simulink model "CSI_0313_4DC"  (R2018a)
settings: Solver=FixedStepDiscrete  StartTime=0.0  StopTime=Tstop  FixedStep=Tdelt  MaxStep=1e-4  RelTol=1e-3
values from neighbouring files (symbols this model uses):
  C = 12e-6    (= 1.2e-05)    [Inputparameter.m]
  Cdc = 4.76*10^-3    (= 0.00476)    [Inputparameter.m]
  Cemc = 1.5e-6    (= 1.5e-06)    [Inputparameter.m]
  fanalog = 7000    [Run.m]
  fKIUdc = 6    [Run.m]
  fKPUdc = 0.4    [Run.m]
  fTs = Update/18000    (= 0.000111111111111)    [Run.m]
  K120 = 0.0    (= 0)    [Run.m]
  K21 = 0.0    (= 0)    [Run.m]
  K5 = 0.0    (= 0)    [Run.m]
  K7 = 0.0    (= 0)    [Run.m]
  Kipll = 1.0    (= 1)    [Run.m]
  klmt = 0.3    [Run.m]
  Kpll = 20.0    (= 20)    [Run.m]
  Lgrid = 7.717e-4*10    (= 0.007717)    [Run.m]
  Lline = 60e-6    (= 6e-05)    [Inputparameter.m]
  Lpwm = 184.8e-6    (= 0.0001848)    [Inputparameter.m]
  mode = 1    [Run.m]
  Nsw = 18000/fbase    [Run.m]
  Qbpf = 1.0    (= 1)    [Run.m]
  Rc = 10e-3    (= 0.01)    [Inputparameter.m]
  Remc = 1e-3    (= 0.001)    [Inputparameter.m]
  Rgrid = 2*pi*fbase*Lgrid/XR    [Run.m]
  Rline = 4.95e-3    (= 0.00495)    [Inputparameter.m]
  Rpre = 2.2    [Inputparameter.m]
  Rpwm = 6.2e-3    (= 0.0062)    [Inputparameter.m]
  Tdelt = (fTs)/(200*Update)    (= 2.77777777778e-07)    [Run.m]
  Tdt = 1.27e-6    (= 1.27e-06)    [Run.m]
  tstart = 0.2    [Run.m]
  Tvstep = 1.5    [Run.m]
  Update = 2    [Run.m]
  Vbase = 400*sqrt(2/3)    [Inputparameter.m]
undefined symbols (not defined in the file or in its folder): sigbuilder_block
libraries: powerlib x412
(part 4 of 13)

== system CSI_0313_4DC/AIP2/Subsystem5 ==
  Vabc : Inport
  Trigger : TriggerPort  TriggerType=falling  VariantControl=Variant  PortDimensions=1
  Gain6 : Gain  Gain=1/Vbase
  PLL : Subsystem  mask{fKPPLL=Kpll, fKIPLL=Kipll, fDltMin=-19, fDltMax=19, fFqBase=50, fTs=fTs}
      mask prompts: fKPPLL "PLL Proportional Gain"; fKIPLL "PLL Integral Coefficient"; fDltMin "fDelta Minimum Limitation [rad/s]"; fDltMax "fDelta Maximum Limitation [rad/s]"; fFqBase "Base Frequency [Hz]"; fTs "Sample Time [s]"
  Freq : Outport
  wt : Outport  Port=2
  VdPosPU : Outport  Port=3
  wires:
  Gain6/1 -> [VabcPU]
  PLL/2(wt) -> wt/1
  Vabc/1 -> Gain6/1
  [VabcPU] -> PLL/1(Vabc)
  PLL/3(VdPos) -> VdPosPU/1
  PLL/1(f) -> Freq/1

== system CSI_0313_4DC/AIP2/Subsystem7 ==
  Vpcc : Inport
  Vdcs : Inport  Port=2
  VdcsLP : Inport  Port=3
  "Freq " : Inport  Port=4
  wt : Inport  Port=5
  Enable : EnablePort
  Trigger : TriggerPort  TriggerType=falling  VariantControl=Variant  PortDimensions=1
  ABC_To_RIZ1 : MATLAB Function  TreatAsAtomicUnit=on
  "BPF " : Subsystem
  Gain1 : Gain  Gain=Vbase
  Gain5 : Gain  Gain=1/Vbase
  Pos Compensation1 : Subsystem
  RIZ_To_ABC1 : MATLAB Function  TreatAsAtomicUnit=on
  Scope2 : Scope  NumInputPorts=3
  Scope4 : Scope  NumInputPorts=2
  Subsystem5 : Subsystem
  Sum : Sum
  Vmod : Outport  VectorParamsAs1DForOutWhenUnconnected=on
  wires:
  [VabcBPFPU] -> Sum/2
  Pos Compensation1/1(VabcFBPU) -> [VabcFBPU]
  [wt] -> Pos Compensation1/2(wt)
  [Vdc] -> Pos Compensation1/1(Vdc)
  wt/1 -> [wt], Scope4/2
  "Freq "/1 -> [freq], Scope4/1
  VdcsLP/1 -> [VdcLP]
  Gain5/1 -> [VrizPU]
  [Vriz] -> Gain5/1
  [Vdc] -> Scope2/3
  [VdcLP] -> Subsystem5/2(Vdc)
  Vdcs/1 -> [Vdc]
  [VabcBPFPU] -> Scope2/2
  [VabcFBPU] -> Scope2/1
  Vpcc/1 -> [Vabc]
  [VrizBPFPU] -> RIZ_To_ABC1/1(RIZ)
  ABC_To_RIZ1/1(RIZ) -> [Vriz]
  [Vabc] -> ABC_To_RIZ1/1(ABC)
  [freq] -> "BPF "/2(Freq)
  RIZ_To_ABC1/1(ABC) -> [VabcBPFPU]
  [VrizPU] -> "BPF "/1(Vriz)
  "BPF "/1(VpccBPF) -> [VrizBPFPU]
  [VMod_3rd] -> Vmod/1
  [VabcMod] -> Subsystem5/1(Vabc)
  Gain1/1 -> [VabcMod]
  Sum/1 -> Gain1/1
  Subsystem5/1(Vmod) -> [VMod_3rd]
  [VabcFBPU] -> Sum/1

== system CSI_0313_4DC/AIP3/Cemc ==
  RLemc1 : powerlib/Elements/Series RLC Branch  LConnTagsString=__new0  RConnTagsString=__new0  BranchType=RC  Resistance=Remc  Inductance=Lpwm  SetiL0=off  InitialCurrent=0  Capacitance=Cemc  Setx0=off  InitialVoltage=326.6  Measurements=None
      settings: SourceProductName=Simscape Electrical
  RLemc2 : powerlib/Elements/Series RLC Branch  LConnTagsString=__new0  RConnTagsString=__new0  BranchType=RC  Resistance=Remc  Inductance=Lpwm  SetiL0=off  InitialCurrent=0  Capacitance=Cemc  Setx0=off  InitialVoltage=326.6  Measurements=None
      settings: SourceProductName=Simscape Electrical
  RLemc3 : powerlib/Elements/Series RLC Branch  LConnTagsString=__new0  RConnTagsString=__new0  BranchType=RC  Resistance=Remc  Inductance=Lpwm  SetiL0=off  InitialCurrent=0  Capacitance=Cemc  Setx0=off  InitialVoltage=326.6  Measurements=None
      settings: SourceProductName=Simscape Electrical
  ConnA : PMIOPort  Side=Left
  ConnB : PMIOPort  Port=2  Side=Left
  ConnC : PMIOPort  Port=3  Side=Left
  Gnd : PMIOPort  Port=4  Side=Right
  connections:
  RLemc1/LConn1 -- ConnA/RConn1
  RLemc3/RConn1 -- Gnd/RConn1 -- RLemc1/RConn1 -- RLemc2/RConn1
  RLemc2/LConn1 -- ConnB/RConn1
  RLemc3/LConn1 -- ConnC/RConn1

== system CSI_0313_4DC/AIP3/LCL Output Filter ==
  RL : powerlib/Elements/Series RLC Branch  LConnTagsString=__new0  RConnTagsString=__new0  BranchType=RL  Resistance=Rpwm  Inductance=Lpwm  SetiL0=off  InitialCurrent=0  Capacitance=1e-6  Setx0=off  InitialVoltage=0  Measurements=None
      settings: SourceProductName=Simscape Electrical
  RL1 : powerlib/Elements/Series RLC Branch  LConnTagsString=__new0  RConnTagsString=__new0  BranchType=RL  Resistance=Rpwm  Inductance=Lpwm  SetiL0=off  InitialCurrent=0  Capacitance=1e-6  Setx0=off  InitialVoltage=0  Measurements=None
      settings: SourceProductName=Simscape Electrical
  RL2 : powerlib/Elements/Series RLC Branch  LConnTagsString=__new0  RConnTagsString=__new0  BranchType=RL  Resistance=Rpwm  Inductance=Lpwm  SetiL0=off  InitialCurrent=0  Capacitance=1e-6  Setx0=off  InitialVoltage=0  Measurements=None
      settings: SourceProductName=Simscape Electrical
  RL3 : powerlib/Elements/Series RLC Branch  LConnTagsString=__new0  RConnTagsString=__new0  BranchType=RL  Resistance=Rline  Inductance=Lline  SetiL0=off  InitialCurrent=0  Capacitance=1e-6  Setx0=off  InitialVoltage=0  Measurements=None
      settings: SourceProductName=Simscape Electrical
  RL4 : powerlib/Elements/Series RLC Branch  LConnTagsString=__new0  RConnTagsString=__new0  BranchType=RL  Resistance=Rline  Inductance=Lline  SetiL0=off  InitialCurrent=0  Capacitance=1e-6  Setx0=off  InitialVoltage=0  Measurements=None
      settings: SourceProductName=Simscape Electrical
  RL5 : powerlib/Elements/Series RLC Branch  LConnTagsString=__new0  RConnTagsString=__new0  BranchType=RL  Resistance=Rline  Inductance=Lline  SetiL0=off  InitialCurrent=0  Capacitance=1e-6  Setx0=off  InitialVoltage=0  Measurements=None
      settings: SourceProductName=Simscape Electrical
  RL6 : powerlib/Elements/Series RLC Branch  LConnTagsString=__new0  RConnTagsString=__new0  BranchType=RC  Resistance=Rc  Inductance=Lpwm  SetiL0=off  InitialCurrent=0  Capacitance=C  Setx0=off  InitialVoltage=326.6  Measurements=None
      settings: SourceProductName=Simscape Electrical
  RL7 : powerlib/Elements/Series RLC Branch  LConnTagsString=__new0  RConnTagsString=__new0  BranchType=RC  Resistance=Rc  Inductance=Lpwm  SetiL0=off  InitialCurrent=0  Capacitance=C  Setx0=off  InitialVoltage=326.6  Measurements=None
      settings: SourceProductName=Simscape Electrical
  RL8 : powerlib/Elements/Series RLC Branch  LConnTagsString=__new0  RConnTagsString=__new0  BranchType=RC  Resistance=Rc  Inductance=Lpwm  SetiL0=off  InitialCurrent=0  Capacitance=C  Setx0=off  InitialVoltage=326.6  Measurements=None
      settings: SourceProductName=Simscape Electrical
  ConnA : PMIOPort  Side=Left
  Conna : PMIOPort  Port=2  Side=Right
  ConnB : PMIOPort  Port=3  Side=Left
  Connb : PMIOPort  Port=4  Side=Right
  ConnC : PMIOPort  Port=5  Side=Left
  Connc : PMIOPort  Port=6  Side=Right
  "Neutral " : PMIOPort  Port=7  Side=Right
  connections:
  RL4/LConn1 -- RL7/LConn1 -- RL1/RConn1
  RL/LConn1 -- ConnA/RConn1
  RL3/LConn1 -- RL6/LConn1 -- RL/RConn1
  RL5/LConn1 -- RL8/LConn1 -- RL2/RConn1
  RL4/RConn1 -- Connb/RConn1
  RL6/RConn1 -- RL7/RConn1 -- "Neutral "/RConn1 -- RL8/RConn1
  RL1/LConn1 -- ConnB/RConn1
  RL3/RConn1 -- Conna/RConn1
  RL2/LConn1 -- ConnC/RConn1
  RL5/RConn1 -- Connc/RConn1

== system CSI_0313_4DC/AIP3/RB-IGBT Bridge1 ==
  Gate : Inport
  Demux : Demux
  Demux1 : Demux
  Demux2 : Demux
  Demux3 : Demux  Outputs=3
  IGBT/Diode{1..5,12} (6 alike) : powerlib/Power Electronics/IGBT//Diode  Ron=Ron1  Rs=1e6  Cs=Cout  Measurements=off
      settings: SourceProductName=Simscape Electrical
  IGBT/Diode{6..11} (6 alike) : powerlib/Power Electronics/IGBT//Diode  Ron=Ron2  Rs=1e6  Cs=Cout  Measurements=off
      settings: SourceProductName=Simscape Electrical
  positive : PMIOPort  Tag=PMCPort  Side=Right
  netural : PMIOPort  Tag=PMCPort  Port=2  Side=Right
  negative : PMIOPort  Tag=PMCPort  Port=3  Side=Right
  A : PMIOPort  Tag=PMCPort  Port=4  Side=Left
  B : PMIOPort  Tag=PMCPort  Port=5  Side=Left
  C : PMIOPort  Tag=PMCPort  Port=6  Side=Left
  wires:
  Demux3/3 -> Demux2/1  "PulseC"
  Demux3/2 -> Demux1/1  "PulseB"
  Demux3/1 -> Demux/1  "PulseA"
  [PulseC_2n] -> IGBT/Diode4/1
  Demux2/4 -> [PulseC_2n]
  Demux2/3 -> [PulseC_1n]
  Demux2/2 -> [PulseC_2p]
  Demux2/1 -> [PulseC_1p]
  [PulseB_2n] -> IGBT/Diode3/1
  Demux1/4 -> [PulseB_2n]
  Demux1/3 -> [PulseB_1n]
  [PulseB_2p] -> IGBT/Diode8/1
  Demux1/2 -> [PulseB_2p]
  [PulseB_1p] -> IGBT/Diode1/1
  Demux1/1 -> [PulseB_1p]
  [PulseA_2n] -> IGBT/Diode12/1
  Demux/4 -> [PulseA_2n]
  Demux/3 -> [PulseA_1n]
  [PulseA_2p] -> IGBT/Diode6/1
  Demux/2 -> [PulseA_2p]
  [PulseA_1p] -> IGBT/Diode5/1
  Demux/1 -> [PulseA_1p]
  Gate/1 -> Demux3/1
  [PulseA_1n] -> IGBT/Diode7/1
  [PulseB_1n] -> IGBT/Diode9/1
  [PulseC_2p] -> IGBT/Diode10/1
  [PulseC_1n] -> IGBT/Diode11/1
  [PulseC_1p] -> IGBT/Diode2/1
  connections:
  C/RConn1 -- IGBT/Diode4/LConn1 -- IGBT/Diode2/RConn1 -- IGBT/Diode11/LConn1
  netural/RConn1 -- IGBT/Diode10/LConn1 -- IGBT/Diode8/LConn1 -- IGBT/Diode6/LConn1
  A/RConn1 -- IGBT/Diode12/LConn1 -- IGBT/Diode5/RConn1 -- IGBT/Diode7/LConn1
  B/RConn1 -- IGBT/Diode3/LConn1 -- IGBT/Diode1/RConn1 -- IGBT/Diode9/LConn1
  IGBT/Diode2/LConn1 -- positive/RConn1 -- IGBT/Diode1/LConn1 -- IGBT/Diode5/LConn1
  IGBT/Diode4/RConn1 -- negative/RConn1 -- IGBT/Diode12/RConn1 -- IGBT/Diode3/RConn1
  IGBT/Diode7/RConn1 -- IGBT/Diode6/RConn1
  IGBT/Diode9/RConn1 -- IGBT/Diode8/RConn1
  IGBT/Diode11/RConn1 -- IGBT/Diode10/RConn1

== system CSI_0313_4DC/AIP3/SPWM_Three Level ==
  VMod_3rd : Inport
  Freq : Inport  Port=2
  Tstart : Inport  Port=3
  Carrier Gen : MATLAB Function  TreatAsAtomicUnit=on  mask{fdelt=Tdelt}
      mask prompts: fdelt "Simulation Step [s]"
  Constant1 : Constant  Value=Nsw
  Constant2 : Constant  Value=18000
  Constant3 : Constant  Value=55e-6
  Constant4 : Constant  Value=Update
  Constant6 : Constant  Value=Update
  Delay1 : Delay  DelayLength=1  SampleTime=fTs
  Demux1 : Demux  Outputs=3
  Mux : Mux
  Product1 : Product
  Product2 : Product
  Pulse Modulation : MATLAB Function  TreatAsAtomicUnit=on
  Scope1 : Scope
  Scope2 : Scope  NumInputPorts=5
  Step : Step  Time=tstart  Before=-1  SampleTime=0
  Switch : Switch  Criteria=u2 > Threshold
  Tdt Insert : MATLAB Function  TreatAsAtomicUnit=on  mask{tdt=Tdt, fdelt=Tdelt}
      mask prompts: tdt "Dead Time [s]"; fdelt "Simulation step [s]"
  Voltage update timing generator : MATLAB Function  TreatAsAtomicUnit=on
  Voltage update timing generator1 : MATLAB Function  TreatAsAtomicUnit=on
  Gate : Outport  VectorParamsAs1DForOutWhenUnconnected=on
  Ttrigger : Outport  Port=2  VectorParamsAs1DForOutWhenUnconnected=on
  Ttrigger1 : Outport  Port=3  VectorParamsAs1DForOutWhenUnconnected=on
  chk : Outport  Port=4  VectorParamsAs1DForOutWhenUnconnected=on
  wires:
  Mux/1 -> chk/1
  [chk] -> Mux/4
  [Tupdate] -> Mux/3
  [carrier] -> Mux/1
  Voltage update timing generator/1(Tupdate) -> [Tupdate]
  [Ttrigger] -> Voltage update timing generator/1(Trigger)
  [carrier] -> Pulse Modulation/1(carrier)
  Carrier Gen/1(carrier) -> [carrier]
  Carrier Gen/2(sgn) -> [Ttrigger]
  [Freq] -> Carrier Gen/1(fsw)
  Product2/1 -> Switch/1
  Delay1/1 -> Product2/1
  Constant2/1 -> [Freq], Switch/3
  Constant1/1 -> Product2/2
  Step/1 -> Switch/2
  Freq/1 -> Delay1/1
  [Freq] -> Product1/1
  Product1/1 -> Mux/2
  Constant3/1 -> Product1/2
  Switch/1 -> Scope1/1
  Tstart/1 -> Tdt Insert/2(st)
  [Tupdatex] -> Pulse Modulation/3(update)
  Pulse Modulation/1(Pulse) -> Tdt Insert/1(pulse)
  Constant4/1 -> Voltage update timing generator/2(Update)
  Tdt Insert/1(Gate) -> Gate/1
  Constant6/1 -> Voltage update timing generator1/2(Update)
  [Ttrigger] -> Voltage update timing generator1/1(Trigger)
  [Tupdate] -> Ttrigger1/1
  [Ttrigger] -> Ttrigger/1
  Pulse Modulation/2(chk) -> [chk]
  Voltage update timing generator1/1(Tupdate) -> [Tupdatex]
  [Ttrigger] -> Pulse Modulation/2(sgn)
  VMod_3rd/1 -> [VMod_3rd]
  [VMod_3rd] -> Pulse Modulation/4(mod)
  Pulse Modulation/3(chk1) -> [chk1]
  [Tupdatex] -> Scope2/1
  [Ttrigger] -> Scope2/2
  [VMod_3rd] -> Demux1/1
  Demux1/1 -> Scope2/5
  [chk1] -> Scope2/4
  [Tupdate] -> Scope2/3

== system CSI_0313_4DC/AIP3/Subsystem ==
  In1 : Inport
  Demux2 : Demux  Outputs=3
  IIR_1st1 : MATLAB Function  TreatAsAtomicUnit=on  mask{fc=fanalog, fTs=Tdelt}
      mask prompts: fc "Cut-off frequency [Hz]"; fTs "Sample time [s]"
      mask help: 1st-order Low Pass Filter
  IIR_1st2 : MATLAB Function  TreatAsAtomicUnit=on  mask{fc=fanalog, fTs=Tdelt}
      mask prompts: fc "Cut-off frequency [Hz]"; fTs "Sample time [s]"
      mask help: 1st-order Low Pass Filter
  IIR_1st3 : MATLAB Function  TreatAsAtomicUnit=on  mask{fc=fanalog, fTs=Tdelt}
      mask prompts: fc "Cut-off frequency [Hz]"; fTs "Sample time [s]"
      mask help: 1st-order Low Pass Filter
  Mux1 : Mux  Inputs=3
  Out1 : Outport  VectorParamsAs1DForOutWhenUnconnected=on
  wires:
  IIR_1st2/1(y) -> Mux1/2
  In1/1 -> Demux2/1
  Demux2/1 -> IIR_1st1/1(u)
  Demux2/3 -> IIR_1st3/1(u)
  Demux2/2 -> IIR_1st2/1(u)
  IIR_1st3/1(y) -> Mux1/3
  Mux1/1 -> Out1/1
  IIR_1st1/1(y) -> Mux1/1

== system CSI_0313_4DC/AIP3/Subsystem3 ==
  In1 : Inport
  Trigger : TriggerPort  VariantControl=Variant  PortDimensions=1
  IIR_1st1 : MATLAB Function  TreatAsAtomicUnit=on  mask{fc=10, fTs=fTs}
      mask prompts: fc "Cut-off frequency [Hz]"; fTs "Sample time [s]"
      mask help: 1st-order Low Pass Filter
  Out1 : Outport  VectorParamsAs1DForOutWhenUnconnected=on
  wires:
  IIR_1st1/1(y) -> Out1/1
  In1/1 -> IIR_1st1/1(u)

== system CSI_0313_4DC/AIP3/Subsystem5 ==
  Vabc : Inport
  Trigger : TriggerPort  TriggerType=falling  VariantControl=Variant  PortDimensions=1
  Gain6 : Gain  Gain=1/Vbase
  PLL : Subsystem  mask{fKPPLL=Kpll, fKIPLL=Kipll, fDltMin=-19, fDltMax=19, fFqBase=50, fTs=fTs}
      mask prompts: fKPPLL "PLL Proportional Gain"; fKIPLL "PLL Integral Coefficient"; fDltMin "fDelta Minimum Limitation [rad/s]"; fDltMax "fDelta Maximum Limitation [rad/s]"; fFqBase "Base Frequency [Hz]"; fTs "Sample Time [s]"
  Freq : Outport
  wt : Outport  Port=2
  VdPosPU : Outport  Port=3
  wires:
  PLL/1(f) -> Freq/1
  PLL/3(VdPos) -> VdPosPU/1
  [VabcPU] -> PLL/1(Vabc)
  Vabc/1 -> Gain6/1
  PLL/2(wt) -> wt/1
  Gain6/1 -> [VabcPU]

== system CSI_0313_4DC/AIP3/Subsystem7 ==
  Vpcc : Inport
  Vdcs : Inport  Port=2
  VdcsLP : Inport  Port=3
  "Freq " : Inport  Port=4
  wt : Inport  Port=5
  Enable : EnablePort
  Trigger : TriggerPort  TriggerType=falling  VariantControl=Variant  PortDimensions=1
  ABC_To_RIZ1 : MATLAB Function  TreatAsAtomicUnit=on
  "BPF " : Subsystem
  Gain1 : Gain  Gain=Vbase
  Gain5 : Gain  Gain=1/Vbase
  Pos Compensation1 : Subsystem
  RIZ_To_ABC1 : MATLAB Function  TreatAsAtomicUnit=on
  Scope2 : Scope  NumInputPorts=3
  Scope4 : Scope  NumInputPorts=2
  Subsystem5 : Subsystem
  Sum : Sum
  Vmod : Outport  VectorParamsAs1DForOutWhenUnconnected=on
  wires:
  [VabcFBPU] -> Sum/1
  Subsystem5/1(Vmod) -> [VMod_3rd]
  Sum/1 -> Gain1/1
  Gain1/1 -> [VabcMod]
  [VabcMod] -> Subsystem5/1(Vabc)
  [VMod_3rd] -> Vmod/1
  "BPF "/1(VpccBPF) -> [VrizBPFPU]
  [VrizPU] -> "BPF "/1(Vriz)
  RIZ_To_ABC1/1(ABC) -> [VabcBPFPU]
  [freq] -> "BPF "/2(Freq)
  [Vabc] -> ABC_To_RIZ1/1(ABC)
  ABC_To_RIZ1/1(RIZ) -> [Vriz]
  [VrizBPFPU] -> RIZ_To_ABC1/1(RIZ)
  Vpcc/1 -> [Vabc]
  [VabcFBPU] -> Scope2/1
  [VabcBPFPU] -> Scope2/2
  Vdcs/1 -> [Vdc]
  [VdcLP] -> Subsystem5/2(Vdc)
  [Vdc] -> Scope2/3
  [Vriz] -> Gain5/1
  Gain5/1 -> [VrizPU]
  VdcsLP/1 -> [VdcLP]
  "Freq "/1 -> Scope4/1, [freq]
  wt/1 -> Scope4/2, [wt]
  [Vdc] -> Pos Compensation1/1(Vdc)
  [wt] -> Pos Compensation1/2(wt)
  Pos Compensation1/1(VabcFBPU) -> [VabcFBPU]
  [VabcBPFPU] -> Sum/2

== system CSI_0313_4DC/AIP4/Cemc ==
  RLemc1 : powerlib/Elements/Series RLC Branch  LConnTagsString=__new0  RConnTagsString=__new0  BranchType=RC  Resistance=Remc  Inductance=Lpwm  SetiL0=off  InitialCurrent=0  Capacitance=Cemc  Setx0=off  InitialVoltage=326.6  Measurements=None
      settings: SourceProductName=Simscape Electrical
  RLemc2 : powerlib/Elements/Series RLC Branch  LConnTagsString=__new0  RConnTagsString=__new0  BranchType=RC  Resistance=Remc  Inductance=Lpwm  SetiL0=off  InitialCurrent=0  Capacitance=Cemc  Setx0=off  InitialVoltage=326.6  Measurements=None
      settings: SourceProductName=Simscape Electrical
  RLemc3 : powerlib/Elements/Series RLC Branch  LConnTagsString=__new0  RConnTagsString=__new0  BranchType=RC  Resistance=Remc  Inductance=Lpwm  SetiL0=off  InitialCurrent=0  Capacitance=Cemc  Setx0=off  InitialVoltage=326.6  Measurements=None
      settings: SourceProductName=Simscape Electrical
  ConnA : PMIOPort  Side=Left
  ConnB : PMIOPort  Port=2  Side=Left
  ConnC : PMIOPort  Port=3  Side=Left
  Gnd : PMIOPort  Port=4  Side=Right
  connections:
  RLemc3/LConn1 -- ConnC/RConn1
  RLemc2/LConn1 -- ConnB/RConn1
  RLemc2/RConn1 -- RLemc1/RConn1 -- Gnd/RConn1 -- RLemc3/RConn1
  RLemc1/LConn1 -- ConnA/RConn1

== system CSI_0313_4DC/AIP4/LCL Output Filter ==
  RL : powerlib/Elements/Series RLC Branch  LConnTagsString=__new0  RConnTagsString=__new0  BranchType=RL  Resistance=Rpwm  Inductance=Lpwm  SetiL0=off  InitialCurrent=0  Capacitance=1e-6  Setx0=off  InitialVoltage=0  Measurements=None
      settings: SourceProductName=Simscape Electrical
  RL1 : powerlib/Elements/Series RLC Branch  LConnTagsString=__new0  RConnTagsString=__new0  BranchType=RL  Resistance=Rpwm  Inductance=Lpwm  SetiL0=off  InitialCurrent=0  Capacitance=1e-6  Setx0=off  InitialVoltage=0  Measurements=None
      settings: SourceProductName=Simscape Electrical
  RL2 : powerlib/Elements/Series RLC Branch  LConnTagsString=__new0  RConnTagsString=__new0  BranchType=RL  Resistance=Rpwm  Inductance=Lpwm  SetiL0=off  InitialCurrent=0  Capacitance=1e-6  Setx0=off  InitialVoltage=0  Measurements=None
      settings: SourceProductName=Simscape Electrical
  RL3 : powerlib/Elements/Series RLC Branch  LConnTagsString=__new0  RConnTagsString=__new0  BranchType=RL  Resistance=Rline  Inductance=Lline  SetiL0=off  InitialCurrent=0  Capacitance=1e-6  Setx0=off  InitialVoltage=0  Measurements=None
      settings: SourceProductName=Simscape Electrical
  RL4 : powerlib/Elements/Series RLC Branch  LConnTagsString=__new0  RConnTagsString=__new0  BranchType=RL  Resistance=Rline  Inductance=Lline  SetiL0=off  InitialCurrent=0  Capacitance=1e-6  Setx0=off  InitialVoltage=0  Measurements=None
      settings: SourceProductName=Simscape Electrical
  RL5 : powerlib/Elements/Series RLC Branch  LConnTagsString=__new0  RConnTagsString=__new0  BranchType=RL  Resistance=Rline  Inductance=Lline  SetiL0=off  InitialCurrent=0  Capacitance=1e-6  Setx0=off  InitialVoltage=0  Measurements=None
      settings: SourceProductName=Simscape Electrical
  RL6 : powerlib/Elements/Series RLC Branch  LConnTagsString=__new0  RConnTagsString=__new0  BranchType=RC  Resistance=Rc  Inductance=Lpwm  SetiL0=off  InitialCurrent=0  Capacitance=C  Setx0=off  InitialVoltage=326.6  Measurements=None
      settings: SourceProductName=Simscape Electrical
  RL7 : powerlib/Elements/Series RLC Branch  LConnTagsString=__new0  RConnTagsString=__new0  BranchType=RC  Resistance=Rc  Inductance=Lpwm  SetiL0=off  InitialCurrent=0  Capacitance=C  Setx0=off  InitialVoltage=326.6  Measurements=None
      settings: SourceProductName=Simscape Electrical
  RL8 : powerlib/Elements/Series RLC Branch  LConnTagsString=__new0  RConnTagsString=__new0  BranchType=RC  Resistance=Rc  Inductance=Lpwm  SetiL0=off  InitialCurrent=0  Capacitance=C  Setx0=off  InitialVoltage=326.6  Measurements=None
      settings: SourceProductName=Simscape Electrical
  ConnA : PMIOPort  Side=Left
  Conna : PMIOPort  Port=2  Side=Right
  ConnB : PMIOPort  Port=3  Side=Left
  Connb : PMIOPort  Port=4  Side=Right
  ConnC : PMIOPort  Port=5  Side=Left
  Connc : PMIOPort  Port=6  Side=Right
  "Neutral " : PMIOPort  Port=7  Side=Right
  connections:
  RL5/RConn1 -- Connc/RConn1
  RL2/LConn1 -- ConnC/RConn1
  RL3/RConn1 -- Conna/RConn1
  RL1/LConn1 -- ConnB/RConn1
  RL8/RConn1 -- "Neutral "/RConn1 -- RL7/RConn1 -- RL6/RConn1
  RL4/RConn1 -- Connb/RConn1
  RL2/RConn1 -- RL8/LConn1 -- RL5/LConn1
  RL/RConn1 -- RL6/LConn1 -- RL3/LConn1
  RL/LConn1 -- ConnA/RConn1
  RL1/RConn1 -- RL7/LConn1 -- RL4/LConn1

== system CSI_0313_4DC/AIP4/RB-IGBT Bridge1 ==
  Gate : Inport
  Demux : Demux
  Demux1 : Demux
  Demux2 : Demux
  Demux3 : Demux  Outputs=3
  IGBT/Diode{1..5,12} (6 alike) : powerlib/Power Electronics/IGBT//Diode  Ron=Ron1  Rs=1e6  Cs=Cout  Measurements=off
      settings: SourceProductName=Simscape Electrical
  IGBT/Diode{6..11} (6 alike) : powerlib/Power Electronics/IGBT//Diode  Ron=Ron2  Rs=1e6  Cs=Cout  Measurements=off
      settings: SourceProductName=Simscape Electrical
  positive : PMIOPort  Tag=PMCPort  Side=Right
  netural : PMIOPort  Tag=PMCPort  Port=2  Side=Right
  negative : PMIOPort  Tag=PMCPort  Port=3  Side=Right
  A : PMIOPort  Tag=PMCPort  Port=4  Side=Left
  B : PMIOPort  Tag=PMCPort  Port=5  Side=Left
  C : PMIOPort  Tag=PMCPort  Port=6  Side=Left
  wires:
  [PulseC_1p] -> IGBT/Diode2/1
  [PulseC_1n] -> IGBT/Diode11/1
  [PulseC_2p] -> IGBT/Diode10/1
  [PulseB_1n] -> IGBT/Diode9/1
  [PulseA_1n] -> IGBT/Diode7/1
  Gate/1 -> Demux3/1
  Demux/1 -> [PulseA_1p]
  [PulseA_1p] -> IGBT/Diode5/1
  Demux/2 -> [PulseA_2p]
  [PulseA_2p] -> IGBT/Diode6/1
  Demux/3 -> [PulseA_1n]
  Demux/4 -> [PulseA_2n]
  [PulseA_2n] -> IGBT/Diode12/1
  Demux1/1 -> [PulseB_1p]
  [PulseB_1p] -> IGBT/Diode1/1
  Demux1/2 -> [PulseB_2p]
  [PulseB_2p] -> IGBT/Diode8/1
  Demux1/3 -> [PulseB_1n]
  Demux1/4 -> [PulseB_2n]
  [PulseB_2n] -> IGBT/Diode3/1
  Demux2/1 -> [PulseC_1p]
  Demux2/2 -> [PulseC_2p]
  Demux2/3 -> [PulseC_1n]
  Demux2/4 -> [PulseC_2n]
  [PulseC_2n] -> IGBT/Diode4/1
  Demux3/1 -> Demux/1  "PulseA"
  Demux3/2 -> Demux1/1  "PulseB"
  Demux3/3 -> Demux2/1  "PulseC"
  connections:
  IGBT/Diode11/RConn1 -- IGBT/Diode10/RConn1
  IGBT/Diode9/RConn1 -- IGBT/Diode8/RConn1
  IGBT/Diode7/RConn1 -- IGBT/Diode6/RConn1
  IGBT/Diode3/RConn1 -- IGBT/Diode12/RConn1 -- negative/RConn1 -- IGBT/Diode4/RConn1
  IGBT/Diode5/LConn1 -- IGBT/Diode1/LConn1 -- positive/RConn1 -- IGBT/Diode2/LConn1
  IGBT/Diode9/LConn1 -- IGBT/Diode1/RConn1 -- IGBT/Diode3/LConn1 -- B/RConn1
  IGBT/Diode7/LConn1 -- IGBT/Diode5/RConn1 -- IGBT/Diode12/LConn1 -- A/RConn1
  IGBT/Diode6/LConn1 -- IGBT/Diode8/LConn1 -- IGBT/Diode10/LConn1 -- netural/RConn1
  IGBT/Diode11/LConn1 -- IGBT/Diode2/RConn1 -- IGBT/Diode4/LConn1 -- C/RConn1

== system CSI_0313_4DC/AIP4/SPWM_Three Level ==
  VMod_3rd : Inport
  Freq : Inport  Port=2
  Tstart : Inport  Port=3
  Carrier Gen : MATLAB Function  TreatAsAtomicUnit=on  mask{fdelt=Tdelt}
      mask prompts: fdelt "Simulation Step [s]"
  Constant1 : Constant  Value=Nsw
  Constant2 : Constant  Value=18000
  Constant3 : Constant  Value=55e-6
  Constant4 : Constant  Value=Update
  Constant6 : Constant  Value=Update
  Delay1 : Delay  DelayLength=1  SampleTime=fTs
  Demux1 : Demux  Outputs=3
  Mux : Mux
  Product1 : Product
  Product2 : Product
  Pulse Modulation : MATLAB Function  TreatAsAtomicUnit=on
  Scope1 : Scope
  Scope2 : Scope  NumInputPorts=5
  Step : Step  Time=tstart  Before=-1  SampleTime=0
  Switch : Switch  Criteria=u2 > Threshold
  Tdt Insert : MATLAB Function  TreatAsAtomicUnit=on  mask{tdt=Tdt, fdelt=Tdelt}
      mask prompts: tdt "Dead Time [s]"; fdelt "Simulation step [s]"
  Voltage update timing generator : MATLAB Function  TreatAsAtomicUnit=on
  Voltage update timing generator1 : MATLAB Function  TreatAsAtomicUnit=on
  Gate : Outport  VectorParamsAs1DForOutWhenUnconnected=on
  Ttrigger : Outport  Port=2  VectorParamsAs1DForOutWhenUnconnected=on
  Ttrigger1 : Outport  Port=3  VectorParamsAs1DForOutWhenUnconnected=on
  chk : Outport  Port=4  VectorParamsAs1DForOutWhenUnconnected=on
  wires:
  [Tupdate] -> Scope2/3
  [chk1] -> Scope2/4
  Demux1/1 -> Scope2/5
  [VMod_3rd] -> Demux1/1
  [Ttrigger] -> Scope2/2
  [Tupdatex] -> Scope2/1
  Pulse Modulation/3(chk1) -> [chk1]
  [VMod_3rd] -> Pulse Modulation/4(mod)
  VMod_3rd/1 -> [VMod_3rd]
  [Ttrigger] -> Pulse Modulation/2(sgn)
  Voltage update timing generator1/1(Tupdate) -> [Tupdatex]
  Pulse Modulation/2(chk) -> [chk]
  [Ttrigger] -> Ttrigger/1
  [Tupdate] -> Ttrigger1/1
  [Ttrigger] -> Voltage update timing generator1/1(Trigger)
  Constant6/1 -> Voltage update timing generator1/2(Update)
  Tdt Insert/1(Gate) -> Gate/1
  Constant4/1 -> Voltage update timing generator/2(Update)
  Pulse Modulation/1(Pulse) -> Tdt Insert/1(pulse)
  [Tupdatex] -> Pulse Modulation/3(update)
  Tstart/1 -> Tdt Insert/2(st)
  Switch/1 -> Scope1/1
  Constant3/1 -> Product1/2
  Product1/1 -> Mux/2
  [Freq] -> Product1/1
  Freq/1 -> Delay1/1
  Step/1 -> Switch/2
  Constant1/1 -> Product2/2
  Constant2/1 -> Switch/3, [Freq]
  Delay1/1 -> Product2/1
  Product2/1 -> Switch/1
  [Freq] -> Carrier Gen/1(fsw)
  Carrier Gen/2(sgn) -> [Ttrigger]
  Carrier Gen/1(carrier) -> [carrier]
  [carrier] -> Pulse Modulation/1(carrier)
  [Ttrigger] -> Voltage update timing generator/1(Trigger)
  Voltage update timing generator/1(Tupdate) -> [Tupdate]
  [carrier] -> Mux/1
  [Tupdate] -> Mux/3
  [chk] -> Mux/4
  Mux/1 -> chk/1

== system CSI_0313_4DC/AIP4/Subsystem ==
  In1 : Inport
  Demux2 : Demux  Outputs=3
  IIR_1st1 : MATLAB Function  TreatAsAtomicUnit=on  mask{fc=fanalog, fTs=Tdelt}
      mask prompts: fc "Cut-off frequency [Hz]"; fTs "Sample time [s]"
      mask help: 1st-order Low Pass Filter
  IIR_1st2 : MATLAB Function  TreatAsAtomicUnit=on  mask{fc=fanalog, fTs=Tdelt}
      mask prompts: fc "Cut-off frequency [Hz]"; fTs "Sample time [s]"
      mask help: 1st-order Low Pass Filter
  IIR_1st3 : MATLAB Function  TreatAsAtomicUnit=on  mask{fc=fanalog, fTs=Tdelt}
      mask prompts: fc "Cut-off frequency [Hz]"; fTs "Sample time [s]"
      mask help: 1st-order Low Pass Filter
  Mux1 : Mux  Inputs=3
  Out1 : Outport  VectorParamsAs1DForOutWhenUnconnected=on
  wires:
  IIR_1st2/1(y) -> Mux1/2
  In1/1 -> Demux2/1
  Demux2/1 -> IIR_1st1/1(u)
  Demux2/3 -> IIR_1st3/1(u)
  Demux2/2 -> IIR_1st2/1(u)
  IIR_1st3/1(y) -> Mux1/3
  Mux1/1 -> Out1/1
  IIR_1st1/1(y) -> Mux1/1

== system CSI_0313_4DC/AIP4/Subsystem3 ==
  In1 : Inport
  Trigger : TriggerPort  VariantControl=Variant  PortDimensions=1
  IIR_1st1 : MATLAB Function  TreatAsAtomicUnit=on  mask{fc=10, fTs=fTs}
      mask prompts: fc "Cut-off frequency [Hz]"; fTs "Sample time [s]"
      mask help: 1st-order Low Pass Filter
  Out1 : Outport  VectorParamsAs1DForOutWhenUnconnected=on
  wires:
  In1/1 -> IIR_1st1/1(u)
  IIR_1st1/1(y) -> Out1/1

== system CSI_0313_4DC/AIP4/Subsystem5 ==
  Vabc : Inport
  Trigger : TriggerPort  TriggerType=falling  VariantControl=Variant  PortDimensions=1
  Gain6 : Gain  Gain=1/Vbase
  PLL : Subsystem  mask{fKPPLL=Kpll, fKIPLL=Kipll, fDltMin=-19, fDltMax=19, fFqBase=50, fTs=fTs}
      mask prompts: fKPPLL "PLL Proportional Gain"; fKIPLL "PLL Integral Coefficient"; fDltMin "fDelta Minimum Limitation [rad/s]"; fDltMax "fDelta Maximum Limitation [rad/s]"; fFqBase "Base Frequency [Hz]"; fTs "Sample Time [s]"
  Freq : Outport
  wt : Outport  Port=2
  VdPosPU : Outport  Port=3
  wires:
  Gain6/1 -> [VabcPU]
  PLL/2(wt) -> wt/1
  Vabc/1 -> Gain6/1
  [VabcPU] -> PLL/1(Vabc)
  PLL/3(VdPos) -> VdPosPU/1
  PLL/1(f) -> Freq/1

== system CSI_0313_4DC/AIP4/Subsystem7 ==
  Vpcc : Inport
  Vdcs : Inport  Port=2
  VdcsLP : Inport  Port=3
  "Freq " : Inport  Port=4
  wt : Inport  Port=5
  Enable : EnablePort
  Trigger : TriggerPort  TriggerType=falling  VariantControl=Variant  PortDimensions=1
  ABC_To_RIZ1 : MATLAB Function  TreatAsAtomicUnit=on
  "BPF " : Subsystem
  Gain1 : Gain  Gain=Vbase
  Gain5 : Gain  Gain=1/Vbase
  Pos Compensation1 : Subsystem
  RIZ_To_ABC1 : MATLAB Function  TreatAsAtomicUnit=on
  Scope2 : Scope  NumInputPorts=3
  Scope4 : Scope  NumInputPorts=2
  Subsystem5 : Subsystem
  Sum : Sum
  Vmod : Outport  VectorParamsAs1DForOutWhenUnconnected=on
  wires:
  [VabcBPFPU] -> Sum/2
  Pos Compensation1/1(VabcFBPU) -> [VabcFBPU]
  [wt] -> Pos Compensation1/2(wt)
  [Vdc] -> Pos Compensation1/1(Vdc)
  wt/1 -> [wt], Scope4/2
  "Freq "/1 -> [freq], Scope4/1
  VdcsLP/1 -> [VdcLP]
  Gain5/1 -> [VrizPU]
  [Vriz] -> Gain5/1
  [Vdc] -> Scope2/3
  [VdcLP] -> Subsystem5/2(Vdc)
  Vdcs/1 -> [Vdc]
  [VabcBPFPU] -> Scope2/2
  [VabcFBPU] -> Scope2/1
  Vpcc/1 -> [Vabc]
  [VrizBPFPU] -> RIZ_To_ABC1/1(RIZ)
  ABC_To_RIZ1/1(RIZ) -> [Vriz]
  [Vabc] -> ABC_To_RIZ1/1(ABC)
  [freq] -> "BPF "/2(Freq)
  RIZ_To_ABC1/1(ABC) -> [VabcBPFPU]
  [VrizPU] -> "BPF "/1(Vriz)
  "BPF "/1(VpccBPF) -> [VrizBPFPU]
  [VMod_3rd] -> Vmod/1
  [VabcMod] -> Subsystem5/1(Vabc)
  Gain1/1 -> [VabcMod]
  Sum/1 -> Gain1/1
  Subsystem5/1(Vmod) -> [VMod_3rd]
  [VabcFBPU] -> Sum/1

== system CSI_0313_4DC/AIP5/Cemc ==
  RLemc1 : powerlib/Elements/Series RLC Branch  LConnTagsString=__new0  RConnTagsString=__new0  BranchType=RC  Resistance=Remc  Inductance=Lpwm  SetiL0=off  InitialCurrent=0  Capacitance=Cemc  Setx0=off  InitialVoltage=326.6  Measurements=None
      settings: SourceProductName=Simscape Electrical
  RLemc2 : powerlib/Elements/Series RLC Branch  LConnTagsString=__new0  RConnTagsString=__new0  BranchType=RC  Resistance=Remc  Inductance=Lpwm  SetiL0=off  InitialCurrent=0  Capacitance=Cemc  Setx0=off  InitialVoltage=326.6  Measurements=None
      settings: SourceProductName=Simscape Electrical
  RLemc3 : powerlib/Elements/Series RLC Branch  LConnTagsString=__new0  RConnTagsString=__new0  BranchType=RC  Resistance=Remc  Inductance=Lpwm  SetiL0=off  InitialCurrent=0  Capacitance=Cemc  Setx0=off  InitialVoltage=326.6  Measurements=None
      settings: SourceProductName=Simscape Electrical
  ConnA : PMIOPort  Side=Left
  ConnB : PMIOPort  Port=2  Side=Left
  ConnC : PMIOPort  Port=3  Side=Left
  Gnd : PMIOPort  Port=4  Side=Right
  connections:
  RLemc1/LConn1 -- ConnA/RConn1
  RLemc3/RConn1 -- Gnd/RConn1 -- RLemc1/RConn1 -- RLemc2/RConn1
  RLemc2/LConn1 -- ConnB/RConn1
  RLemc3/LConn1 -- ConnC/RConn1

== system CSI_0313_4DC/AIP5/LCL Output Filter ==
  RL : powerlib/Elements/Series RLC Branch  LConnTagsString=__new0  RConnTagsString=__new0  BranchType=RL  Resistance=Rpwm  Inductance=Lpwm  SetiL0=off  InitialCurrent=0  Capacitance=1e-6  Setx0=off  InitialVoltage=0  Measurements=None
      settings: SourceProductName=Simscape Electrical
  RL1 : powerlib/Elements/Series RLC Branch  LConnTagsString=__new0  RConnTagsString=__new0  BranchType=RL  Resistance=Rpwm  Inductance=Lpwm  SetiL0=off  InitialCurrent=0  Capacitance=1e-6  Setx0=off  InitialVoltage=0  Measurements=None
      settings: SourceProductName=Simscape Electrical
  RL2 : powerlib/Elements/Series RLC Branch  LConnTagsString=__new0  RConnTagsString=__new0  BranchType=RL  Resistance=Rpwm  Inductance=Lpwm  SetiL0=off  InitialCurrent=0  Capacitance=1e-6  Setx0=off  InitialVoltage=0  Measurements=None
      settings: SourceProductName=Simscape Electrical
  RL3 : powerlib/Elements/Series RLC Branch  LConnTagsString=__new0  RConnTagsString=__new0  BranchType=RL  Resistance=Rline  Inductance=Lline  SetiL0=off  InitialCurrent=0  Capacitance=1e-6  Setx0=off  InitialVoltage=0  Measurements=None
      settings: SourceProductName=Simscape Electrical
  RL4 : powerlib/Elements/Series RLC Branch  LConnTagsString=__new0  RConnTagsString=__new0  BranchType=RL  Resistance=Rline  Inductance=Lline  SetiL0=off  InitialCurrent=0  Capacitance=1e-6  Setx0=off  InitialVoltage=0  Measurements=None
      settings: SourceProductName=Simscape Electrical
  RL5 : powerlib/Elements/Series RLC Branch  LConnTagsString=__new0  RConnTagsString=__new0  BranchType=RL  Resistance=Rline  Inductance=Lline  SetiL0=off  InitialCurrent=0  Capacitance=1e-6  Setx0=off  InitialVoltage=0  Measurements=None
      settings: SourceProductName=Simscape Electrical
  RL6 : powerlib/Elements/Series RLC Branch  LConnTagsString=__new0  RConnTagsString=__new0  BranchType=RC  Resistance=Rc  Inductance=Lpwm  SetiL0=off  InitialCurrent=0  Capacitance=C  Setx0=off  InitialVoltage=326.6  Measurements=None
      settings: SourceProductName=Simscape Electrical
  RL7 : powerlib/Elements/Series RLC Branch  LConnTagsString=__new0  RConnTagsString=__new0  BranchType=RC  Resistance=Rc  Inductance=Lpwm  SetiL0=off  InitialCurrent=0  Capacitance=C  Setx0=off  InitialVoltage=326.6  Measurements=None
      settings: SourceProductName=Simscape Electrical
  RL8 : powerlib/Elements/Series RLC Branch  LConnTagsString=__new0  RConnTagsString=__new0  BranchType=RC  Resistance=Rc  Inductance=Lpwm  SetiL0=off  InitialCurrent=0  Capacitance=C  Setx0=off  InitialVoltage=326.6  Measurements=None
      settings: SourceProductName=Simscape Electrical
  ConnA : PMIOPort  Side=Left
  Conna : PMIOPort  Port=2  Side=Right
  ConnB : PMIOPort  Port=3  Side=Left
  Connb : PMIOPort  Port=4  Side=Right
  ConnC : PMIOPort  Port=5  Side=Left
  Connc : PMIOPort  Port=6  Side=Right
  "Neutral " : PMIOPort  Port=7  Side=Right
  connections:
  RL4/LConn1 -- RL7/LConn1 -- RL1/RConn1
  RL/LConn1 -- ConnA/RConn1
  RL3/LConn1 -- RL6/LConn1 -- RL/RConn1
  RL5/LConn1 -- RL8/LConn1 -- RL2/RConn1
  RL4/RConn1 -- Connb/RConn1
  RL6/RConn1 -- RL7/RConn1 -- "Neutral "/RConn1 -- RL8/RConn1
  RL1/LConn1 -- ConnB/RConn1
  RL3/RConn1 -- Conna/RConn1
  RL2/LConn1 -- ConnC/RConn1
  RL5/RConn1 -- Connc/RConn1

== system CSI_0313_4DC/AIP5/RB-IGBT Bridge1 ==
  Gate : Inport
  Demux : Demux
  Demux1 : Demux
  Demux2 : Demux
  Demux3 : Demux  Outputs=3
  IGBT/Diode{1..5,12} (6 alike) : powerlib/Power Electronics/IGBT//Diode  Ron=Ron1  Rs=1e6  Cs=Cout  Measurements=off
      settings: SourceProductName=Simscape Electrical
  IGBT/Diode{6..11} (6 alike) : powerlib/Power Electronics/IGBT//Diode  Ron=Ron2  Rs=1e6  Cs=Cout  Measurements=off
      settings: SourceProductName=Simscape Electrical
  positive : PMIOPort  Tag=PMCPort  Side=Right
  netural : PMIOPort  Tag=PMCPort  Port=2  Side=Right
  negative : PMIOPort  Tag=PMCPort  Port=3  Side=Right
  A : PMIOPort  Tag=PMCPort  Port=4  Side=Left
  B : PMIOPort  Tag=PMCPort  Port=5  Side=Left
  C : PMIOPort  Tag=PMCPort  Port=6  Side=Left
  wires:
  Demux3/3 -> Demux2/1  "PulseC"
  Demux3/2 -> Demux1/1  "PulseB"
  Demux3/1 -> Demux/1  "PulseA"
  [PulseC_2n] -> IGBT/Diode4/1
  Demux2/4 -> [PulseC_2n]
  Demux2/3 -> [PulseC_1n]
  Demux2/2 -> [PulseC_2p]
  Demux2/1 -> [PulseC_1p]
  [PulseB_2n] -> IGBT/Diode3/1
  Demux1/4 -> [PulseB_2n]
  Demux1/3 -> [PulseB_1n]
  [PulseB_2p] -> IGBT/Diode8/1
  Demux1/2 -> [PulseB_2p]
  [PulseB_1p] -> IGBT/Diode1/1
  Demux1/1 -> [PulseB_1p]
  [PulseA_2n] -> IGBT/Diode12/1
  Demux/4 -> [PulseA_2n]
  Demux/3 -> [PulseA_1n]
  [PulseA_2p] -> IGBT/Diode6/1
  Demux/2 -> [PulseA_2p]
  [PulseA_1p] -> IGBT/Diode5/1
  Demux/1 -> [PulseA_1p]
  Gate/1 -> Demux3/1
  [PulseA_1n] -> IGBT/Diode7/1
  [PulseB_1n] -> IGBT/Diode9/1
  [PulseC_2p] -> IGBT/Diode10/1
  [PulseC_1n] -> IGBT/Diode11/1
  [PulseC_1p] -> IGBT/Diode2/1
  connections:
  C/RConn1 -- IGBT/Diode4/LConn1 -- IGBT/Diode2/RConn1 -- IGBT/Diode11/LConn1
  netural/RConn1 -- IGBT/Diode10/LConn1 -- IGBT/Diode8/LConn1 -- IGBT/Diode6/LConn1
  A/RConn1 -- IGBT/Diode12/LConn1 -- IGBT/Diode5/RConn1 -- IGBT/Diode7/LConn1
  B/RConn1 -- IGBT/Diode3/LConn1 -- IGBT/Diode1/RConn1 -- IGBT/Diode9/LConn1
  IGBT/Diode2/LConn1 -- positive/RConn1 -- IGBT/Diode1/LConn1 -- IGBT/Diode5/LConn1
  IGBT/Diode4/RConn1 -- negative/RConn1 -- IGBT/Diode12/RConn1 -- IGBT/Diode3/RConn1
  IGBT/Diode7/RConn1 -- IGBT/Diode6/RConn1
  IGBT/Diode9/RConn1 -- IGBT/Diode8/RConn1
  IGBT/Diode11/RConn1 -- IGBT/Diode10/RConn1

== system CSI_0313_4DC/AIP5/SPWM_Three Level ==
  VMod_3rd : Inport
  Freq : Inport  Port=2
  Tstart : Inport  Port=3
  Carrier Gen : MATLAB Function  TreatAsAtomicUnit=on  mask{fdelt=Tdelt}
      mask prompts: fdelt "Simulation Step [s]"
  Constant1 : Constant  Value=Nsw
  Constant2 : Constant  Value=18000
  Constant3 : Constant  Value=55e-6
  Constant4 : Constant  Value=Update
  Constant6 : Constant  Value=Update
  Delay1 : Delay  DelayLength=1  SampleTime=fTs
  Demux1 : Demux  Outputs=3
  Mux : Mux
  Product1 : Product
  Product2 : Product
  Pulse Modulation : MATLAB Function  TreatAsAtomicUnit=on
  Scope1 : Scope
  Scope2 : Scope  NumInputPorts=5
  Step : Step  Time=tstart  Before=-1  SampleTime=0
  Switch : Switch  Criteria=u2 > Threshold
  Tdt Insert : MATLAB Function  TreatAsAtomicUnit=on  mask{tdt=Tdt, fdelt=Tdelt}
      mask prompts: tdt "Dead Time [s]"; fdelt "Simulation step [s]"
  Voltage update timing generator : MATLAB Function  TreatAsAtomicUnit=on
  Voltage update timing generator1 : MATLAB Function  TreatAsAtomicUnit=on
  Gate : Outport  VectorParamsAs1DForOutWhenUnconnected=on
  Ttrigger : Outport  Port=2  VectorParamsAs1DForOutWhenUnconnected=on
  Ttrigger1 : Outport  Port=3  VectorParamsAs1DForOutWhenUnconnected=on
  chk : Outport  Port=4  VectorParamsAs1DForOutWhenUnconnected=on
  wires:
  Mux/1 -> chk/1
  [chk] -> Mux/4
  [Tupdate] -> Mux/3
  [carrier] -> Mux/1
  Voltage update timing generator/1(Tupdate) -> [Tupdate]
  [Ttrigger] -> Voltage update timing generator/1(Trigger)
  [carrier] -> Pulse Modulation/1(carrier)
  Carrier Gen/1(carrier) -> [carrier]
  Carrier Gen/2(sgn) -> [Ttrigger]
  [Freq] -> Carrier Gen/1(fsw)
  Product2/1 -> Switch/1
  Delay1/1 -> Product2/1
  Constant2/1 -> [Freq], Switch/3
  Constant1/1 -> Product2/2
  Step/1 -> Switch/2
  Freq/1 -> Delay1/1
  [Freq] -> Product1/1
  Product1/1 -> Mux/2
  Constant3/1 -> Product1/2
  Switch/1 -> Scope1/1
  Tstart/1 -> Tdt Insert/2(st)
  [Tupdatex] -> Pulse Modulation/3(update)
  Pulse Modulation/1(Pulse) -> Tdt Insert/1(pulse)
  Constant4/1 -> Voltage update timing generator/2(Update)
  Tdt Insert/1(Gate) -> Gate/1
  Constant6/1 -> Voltage update timing generator1/2(Update)
  [Ttrigger] -> Voltage update timing generator1/1(Trigger)
  [Tupdate] -> Ttrigger1/1
  [Ttrigger] -> Ttrigger/1
  Pulse Modulation/2(chk) -> [chk]
  Voltage update timing generator1/1(Tupdate) -> [Tupdatex]
  [Ttrigger] -> Pulse Modulation/2(sgn)
  VMod_3rd/1 -> [VMod_3rd]
  [VMod_3rd] -> Pulse Modulation/4(mod)
  Pulse Modulation/3(chk1) -> [chk1]
  [Tupdatex] -> Scope2/1
  [Ttrigger] -> Scope2/2
  [VMod_3rd] -> Demux1/1
  Demux1/1 -> Scope2/5
  [chk1] -> Scope2/4
  [Tupdate] -> Scope2/3

== system CSI_0313_4DC/AIP5/Subsystem ==
  In1 : Inport
  Demux2 : Demux  Outputs=3
  IIR_1st1 : MATLAB Function  TreatAsAtomicUnit=on  mask{fc=fanalog, fTs=Tdelt}
      mask prompts: fc "Cut-off frequency [Hz]"; fTs "Sample time [s]"
      mask help: 1st-order Low Pass Filter
  IIR_1st2 : MATLAB Function  TreatAsAtomicUnit=on  mask{fc=fanalog, fTs=Tdelt}
      mask prompts: fc "Cut-off frequency [Hz]"; fTs "Sample time [s]"
      mask help: 1st-order Low Pass Filter
  IIR_1st3 : MATLAB Function  TreatAsAtomicUnit=on  mask{fc=fanalog, fTs=Tdelt}
      mask prompts: fc "Cut-off frequency [Hz]"; fTs "Sample time [s]"
      mask help: 1st-order Low Pass Filter
  Mux1 : Mux  Inputs=3
  Out1 : Outport  VectorParamsAs1DForOutWhenUnconnected=on
  wires:
  IIR_1st2/1(y) -> Mux1/2
  In1/1 -> Demux2/1
  Demux2/1 -> IIR_1st1/1(u)
  Demux2/3 -> IIR_1st3/1(u)
  Demux2/2 -> IIR_1st2/1(u)
  IIR_1st3/1(y) -> Mux1/3
  Mux1/1 -> Out1/1
  IIR_1st1/1(y) -> Mux1/1

== system CSI_0313_4DC/AIP5/Subsystem3 ==
  In1 : Inport
  Trigger : TriggerPort  VariantControl=Variant  PortDimensions=1
  IIR_1st1 : MATLAB Function  TreatAsAtomicUnit=on  mask{fc=10, fTs=fTs}
      mask prompts: fc "Cut-off frequency [Hz]"; fTs "Sample time [s]"
      mask help: 1st-order Low Pass Filter
  Out1 : Outport  VectorParamsAs1DForOutWhenUnconnected=on
  wires:
  IIR_1st1/1(y) -> Out1/1
  In1/1 -> IIR_1st1/1(u)

== system CSI_0313_4DC/AIP5/Subsystem5 ==
  Vabc : Inport
  Trigger : TriggerPort  TriggerType=falling  VariantControl=Variant  PortDimensions=1
  Gain6 : Gain  Gain=1/Vbase
  PLL : Subsystem  mask{fKPPLL=Kpll, fKIPLL=Kipll, fDltMin=-19, fDltMax=19, fFqBase=50, fTs=fTs}
      mask prompts: fKPPLL "PLL Proportional Gain"; fKIPLL "PLL Integral Coefficient"; fDltMin "fDelta Minimum Limitation [rad/s]"; fDltMax "fDelta Maximum Limitation [rad/s]"; fFqBase "Base Frequency [Hz]"; fTs "Sample Time [s]"
  Freq : Outport
  wt : Outport  Port=2
  VdPosPU : Outport  Port=3
  wires:
  PLL/1(f) -> Freq/1
  PLL/3(VdPos) -> VdPosPU/1
  [VabcPU] -> PLL/1(Vabc)
  Vabc/1 -> Gain6/1
  PLL/2(wt) -> wt/1
  Gain6/1 -> [VabcPU]

== system CSI_0313_4DC/AIP5/Subsystem7 ==
  Vpcc : Inport
  Vdcs : Inport  Port=2
  VdcsLP : Inport  Port=3
  "Freq " : Inport  Port=4
  wt : Inport  Port=5
  Enable : EnablePort
  Trigger : TriggerPort  TriggerType=falling  VariantControl=Variant  PortDimensions=1
  ABC_To_RIZ1 : MATLAB Function  TreatAsAtomicUnit=on
  "BPF " : Subsystem
  Gain1 : Gain  Gain=Vbase
  Gain5 : Gain  Gain=1/Vbase
  Pos Compensation1 : Subsystem
  RIZ_To_ABC1 : MATLAB Function  TreatAsAtomicUnit=on
  Scope2 : Scope  NumInputPorts=3
  Scope4 : Scope  NumInputPorts=2
  Subsystem5 : Subsystem
  Sum : Sum
  Vmod : Outport  VectorParamsAs1DForOutWhenUnconnected=on
  wires:
  [VabcFBPU] -> Sum/1
  Subsystem5/1(Vmod) -> [VMod_3rd]
  Sum/1 -> Gain1/1
  Gain1/1 -> [VabcMod]
  [VabcMod] -> Subsystem5/1(Vabc)
  [VMod_3rd] -> Vmod/1
  "BPF "/1(VpccBPF) -> [VrizBPFPU]
  [VrizPU] -> "BPF "/1(Vriz)
  RIZ_To_ABC1/1(ABC) -> [VabcBPFPU]
  [freq] -> "BPF "/2(Freq)
  [Vabc] -> ABC_To_RIZ1/1(ABC)
  ABC_To_RIZ1/1(RIZ) -> [Vriz]
  [VrizBPFPU] -> RIZ_To_ABC1/1(RIZ)
  Vpcc/1 -> [Vabc]
  [VabcFBPU] -> Scope2/1
  [VabcBPFPU] -> Scope2/2
  Vdcs/1 -> [Vdc]
  [VdcLP] -> Subsystem5/2(Vdc)
  [Vdc] -> Scope2/3
  [Vriz] -> Gain5/1
  Gain5/1 -> [VrizPU]
  VdcsLP/1 -> [VdcLP]
  "Freq "/1 -> Scope4/1, [freq]
  wt/1 -> Scope4/2, [wt]
  [Vdc] -> Pos Compensation1/1(Vdc)
  [wt] -> Pos Compensation1/2(wt)
  Pos Compensation1/1(VabcFBPU) -> [VabcFBPU]
  [VabcBPFPU] -> Sum/2

== system CSI_0313_4DC/AIP6/Cemc ==
  RLemc1 : powerlib/Elements/Series RLC Branch  LConnTagsString=__new0  RConnTagsString=__new0  BranchType=RC  Resistance=Remc  Inductance=Lpwm  SetiL0=off  InitialCurrent=0  Capacitance=Cemc  Setx0=off  InitialVoltage=326.6  Measurements=None
      settings: SourceProductName=Simscape Electrical
  RLemc2 : powerlib/Elements/Series RLC Branch  LConnTagsString=__new0  RConnTagsString=__new0  BranchType=RC  Resistance=Remc  Inductance=Lpwm  SetiL0=off  InitialCurrent=0  Capacitance=Cemc  Setx0=off  InitialVoltage=326.6  Measurements=None
      settings: SourceProductName=Simscape Electrical
  RLemc3 : powerlib/Elements/Series RLC Branch  LConnTagsString=__new0  RConnTagsString=__new0  BranchType=RC  Resistance=Remc  Inductance=Lpwm  SetiL0=off  InitialCurrent=0  Capacitance=Cemc  Setx0=off  InitialVoltage=326.6  Measurements=None
      settings: SourceProductName=Simscape Electrical
  ConnA : PMIOPort  Side=Left
  ConnB : PMIOPort  Port=2  Side=Left
  ConnC : PMIOPort  Port=3  Side=Left
  Gnd : PMIOPort  Port=4  Side=Right
  connections:
  RLemc1/LConn1 -- ConnA/RConn1
  RLemc3/RConn1 -- Gnd/RConn1 -- RLemc1/RConn1 -- RLemc2/RConn1
  RLemc2/LConn1 -- ConnB/RConn1
  RLemc3/LConn1 -- ConnC/RConn1

== system CSI_0313_4DC/AIP6/LCL Output Filter ==
  RL : powerlib/Elements/Series RLC Branch  LConnTagsString=__new0  RConnTagsString=__new0  BranchType=RL  Resistance=Rpwm  Inductance=Lpwm  SetiL0=off  InitialCurrent=0  Capacitance=1e-6  Setx0=off  InitialVoltage=0  Measurements=None
      settings: SourceProductName=Simscape Electrical
  RL1 : powerlib/Elements/Series RLC Branch  LConnTagsString=__new0  RConnTagsString=__new0  BranchType=RL  Resistance=Rpwm  Inductance=Lpwm  SetiL0=off  InitialCurrent=0  Capacitance=1e-6  Setx0=off  InitialVoltage=0  Measurements=None
      settings: SourceProductName=Simscape Electrical
  RL2 : powerlib/Elements/Series RLC Branch  LConnTagsString=__new0  RConnTagsString=__new0  BranchType=RL  Resistance=Rpwm  Inductance=Lpwm  SetiL0=off  InitialCurrent=0  Capacitance=1e-6  Setx0=off  InitialVoltage=0  Measurements=None
      settings: SourceProductName=Simscape Electrical
  RL3 : powerlib/Elements/Series RLC Branch  LConnTagsString=__new0  RConnTagsString=__new0  BranchType=RL  Resistance=Rline  Inductance=Lline  SetiL0=off  InitialCurrent=0  Capacitance=1e-6  Setx0=off  InitialVoltage=0  Measurements=None
      settings: SourceProductName=Simscape Electrical
  RL4 : powerlib/Elements/Series RLC Branch  LConnTagsString=__new0  RConnTagsString=__new0  BranchType=RL  Resistance=Rline  Inductance=Lline  SetiL0=off  InitialCurrent=0  Capacitance=1e-6  Setx0=off  InitialVoltage=0  Measurements=None
      settings: SourceProductName=Simscape Electrical
  RL5 : powerlib/Elements/Series RLC Branch  LConnTagsString=__new0  RConnTagsString=__new0  BranchType=RL  Resistance=Rline  Inductance=Lline  SetiL0=off  InitialCurrent=0  Capacitance=1e-6  Setx0=off  InitialVoltage=0  Measurements=None
      settings: SourceProductName=Simscape Electrical
  RL6 : powerlib/Elements/Series RLC Branch  LConnTagsString=__new0  RConnTagsString=__new0  BranchType=RC  Resistance=Rc  Inductance=Lpwm  SetiL0=off  InitialCurrent=0  Capacitance=C  Setx0=off  InitialVoltage=326.6  Measurements=None
      settings: SourceProductName=Simscape Electrical
  RL7 : powerlib/Elements/Series RLC Branch  LConnTagsString=__new0  RConnTagsString=__new0  BranchType=RC  Resistance=Rc  Inductance=Lpwm  SetiL0=off  InitialCurrent=0  Capacitance=C  Setx0=off  InitialVoltage=326.6  Measurements=None
      settings: SourceProductName=Simscape Electrical
  RL8 : powerlib/Elements/Series RLC Branch  LConnTagsString=__new0  RConnTagsString=__new0  BranchType=RC  Resistance=Rc  Inductance=Lpwm  SetiL0=off  InitialCurrent=0  Capacitance=C  Setx0=off  InitialVoltage=326.6  Measurements=None
      settings: SourceProductName=Simscape Electrical
  ConnA : PMIOPort  Side=Left
  Conna : PMIOPort  Port=2  Side=Right
  ConnB : PMIOPort  Port=3  Side=Left
  Connb : PMIOPort  Port=4  Side=Right
  ConnC : PMIOPort  Port=5  Side=Left
  Connc : PMIOPort  Port=6  Side=Right
  "Neutral " : PMIOPort  Port=7  Side=Right
  connections:
  RL4/LConn1 -- RL7/LConn1 -- RL1/RConn1
  RL/LConn1 -- ConnA/RConn1
  RL3/LConn1 -- RL6/LConn1 -- RL/RConn1
  RL5/LConn1 -- RL8/LConn1 -- RL2/RConn1
  RL4/RConn1 -- Connb/RConn1
  RL6/RConn1 -- RL7/RConn1 -- "Neutral "/RConn1 -- RL8/RConn1
  RL1/LConn1 -- ConnB/RConn1
  RL3/RConn1 -- Conna/RConn1
  RL2/LConn1 -- ConnC/RConn1
  RL5/RConn1 -- Connc/RConn1

== system CSI_0313_4DC/AIP6/RB-IGBT Bridge1 ==
  Gate : Inport
  Demux : Demux
  Demux1 : Demux
  Demux2 : Demux
  Demux3 : Demux  Outputs=3
  IGBT/Diode{1..5,12} (6 alike) : powerlib/Power Electronics/IGBT//Diode  Ron=Ron1  Rs=1e6  Cs=Cout  Measurements=off
      settings: SourceProductName=Simscape Electrical
  IGBT/Diode{6..11} (6 alike) : powerlib/Power Electronics/IGBT//Diode  Ron=Ron2  Rs=1e6  Cs=Cout  Measurements=off
      settings: SourceProductName=Simscape Electrical
  positive : PMIOPort  Tag=PMCPort  Side=Right
  netural : PMIOPort  Tag=PMCPort  Port=2  Side=Right
  negative : PMIOPort  Tag=PMCPort  Port=3  Side=Right
  A : PMIOPort  Tag=PMCPort  Port=4  Side=Left
  B : PMIOPort  Tag=PMCPort  Port=5  Side=Left
  C : PMIOPort  Tag=PMCPort  Port=6  Side=Left
  wires:
  Demux3/3 -> Demux2/1  "PulseC"
  Demux3/2 -> Demux1/1  "PulseB"
  Demux3/1 -> Demux/1  "PulseA"
  [PulseC_2n] -> IGBT/Diode4/1
  Demux2/4 -> [PulseC_2n]
  Demux2/3 -> [PulseC_1n]
  Demux2/2 -> [PulseC_2p]
  Demux2/1 -> [PulseC_1p]
  [PulseB_2n] -> IGBT/Diode3/1
  Demux1/4 -> [PulseB_2n]
  Demux1/3 -> [PulseB_1n]
  [PulseB_2p] -> IGBT/Diode8/1
  Demux1/2 -> [PulseB_2p]
  [PulseB_1p] -> IGBT/Diode1/1
  Demux1/1 -> [PulseB_1p]
  [PulseA_2n] -> IGBT/Diode12/1
  Demux/4 -> [PulseA_2n]
  Demux/3 -> [PulseA_1n]
  [PulseA_2p] -> IGBT/Diode6/1
  Demux/2 -> [PulseA_2p]
  [PulseA_1p] -> IGBT/Diode5/1
  Demux/1 -> [PulseA_1p]
  Gate/1 -> Demux3/1
  [PulseA_1n] -> IGBT/Diode7/1
  [PulseB_1n] -> IGBT/Diode9/1
  [PulseC_2p] -> IGBT/Diode10/1
  [PulseC_1n] -> IGBT/Diode11/1
  [PulseC_1p] -> IGBT/Diode2/1
  connections:
  C/RConn1 -- IGBT/Diode4/LConn1 -- IGBT/Diode2/RConn1 -- IGBT/Diode11/LConn1
  netural/RConn1 -- IGBT/Diode10/LConn1 -- IGBT/Diode8/LConn1 -- IGBT/Diode6/LConn1
  A/RConn1 -- IGBT/Diode12/LConn1 -- IGBT/Diode5/RConn1 -- IGBT/Diode7/LConn1
  B/RConn1 -- IGBT/Diode3/LConn1 -- IGBT/Diode1/RConn1 -- IGBT/Diode9/LConn1
  IGBT/Diode2/LConn1 -- positive/RConn1 -- IGBT/Diode1/LConn1 -- IGBT/Diode5/LConn1
  IGBT/Diode4/RConn1 -- negative/RConn1 -- IGBT/Diode12/RConn1 -- IGBT/Diode3/RConn1
  IGBT/Diode7/RConn1 -- IGBT/Diode6/RConn1
  IGBT/Diode9/RConn1 -- IGBT/Diode8/RConn1
  IGBT/Diode11/RConn1 -- IGBT/Diode10/RConn1
